simulink model "mlf_ifelse"  (R2015b)
settings: Solver=FixedStepDiscrete  SolverMode=SingleTasking  StartTime=0.0  StopTime=1  RelTol=1e-3
PreLoadFcn:
  |  Param1=fi(0.2,1,16,14)
libraries: simulink x1
settings Model: Creator=at-mt  LastModifiedBy=amatsumo
settings DataIOCC: SaveFormat=Array  SignalLoggingSaveFormat=ModelDataLogs  SaveOutput=off  SignalLogging=off  SaveTime=off
settings OptimizationCC: BlockReduction=off  ConditionallyExecuteInputs=off  DefaultParameterBehavior=Inlined  ExpressionDepthLimit=2147483647
settings DebuggingCC: AlgebraicLoopMsg=error  UnderspecifiedInitializationDetection=Classic  MergeDetectMultiDrivingBlocksExec=none  SolverPrmCheckMsg=warning  SingleTaskRateTransMsg=error  FcnCallInpInsideContextMsg=UseLocalSettings  StateNameClashWarn=warning
settings HardwareCC: ProdBitPerPointer=32  ProdLargestAtomicFloat=None  ProdIntDivRoundTo=Undefined  ProdEndianess=Unspecified  ProdWordSize=32  ProdHWDeviceType=ASIC/FPGA->ASIC/FPGA  ProdEqTarget=off
settings GRTTargetCC: GeneratePreprocessorConditionals=Disable all  CombineOutputUpdateFcns=off  GRTInterface=on
settings ConfigComp: CovModelRefEnable=Off  CovSFcnEnable=off

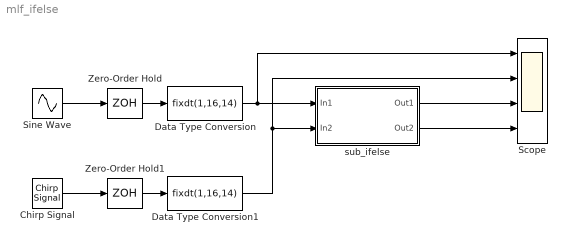
== system mlf_ifelse ==
  Chirp Signal : simulink/Sources/Chirp Signal  f1=10  T=10  f2=500
  Data Type Conversion : DataTypeConversion  OutDataTypeStr=fixdt(1,16,14)
  Data Type Conversion1 : DataTypeConversion  OutDataTypeStr=fixdt(1,16,14)
  Scope : Scope  NumInputPorts=4
  Sine Wave : Sin  Frequency=100  SampleTime=0
  Zero-Order Hold : ZeroOrderHold  SampleTime=1/1000
  Zero-Order Hold1 : ZeroOrderHold  SampleTime=1/1000
  sub_ifelse : Subsystem
  wires:
  Sine Wave/1 -> Zero-Order Hold/1
  Zero-Order Hold/1 -> Data Type Conversion/1
  Data Type Conversion/1 -> sub_ifelse/1(In1), Scope/1
  Chirp Signal/1 -> Zero-Order Hold1/1
  Zero-Order Hold1/1 -> Data Type Conversion1/1
  Data Type Conversion1/1 -> sub_ifelse/2(In2), Scope/2
  sub_ifelse/1(Out1) -> Scope/3
  sub_ifelse/2(Out2) -> Scope/4

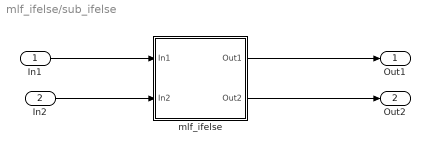
== system mlf_ifelse/sub_ifelse ==
  In1 : Inport
  In2 : Inport  Port=2
  mlf_ifelse : MATLAB Function  TreatAsAtomicUnit=on
  Out1 : Outport
  Out2 : Outport  Port=2
  wires:
  In1/1 -> mlf_ifelse/1(In1)
  mlf_ifelse/1(Out1) -> Out1/1
  In2/1 -> mlf_ifelse/2(In2)
  mlf_ifelse/2(Out2) -> Out2/1

== matlab function mlf_ifelse/sub_ifelse/mlf_ifelse ==
  settings: fimath=hdlfimath;
  data: In1 input; Out1 output; In2 input; Param1 parameter; Out2 output
function [Out1,Out2] = fcn(In1, In2, Param1)
% If Else


% plus
if In1 > Param1
	Out1 = fi(In1 *2 ,1,24,21);
else
	Out1 = fi(0,1,24,21);
end

% if minus, flip wave
if In2 > Param1
	Out2 = fi(In2 * 2,1,24,21);
else
	Out2 = fi(In2 * -2,1,24,21);
end
